simulink model "LQI_MIMO_2017a"  (R2017a)
settings: Solver=VariableStepAuto  StartTime=0.0  StopTime=4  RelTol=1e-3
values from neighbouring files (symbols this model uses):
  Klqi = lqi(sis,Q,R)    [ControladorMotor.m]    (also in ventilador.m = [Klqi Klqi(end)])
  Ts = 0.01    [ventilador.m]
undefined symbols (not defined in the file or in its folder): A, B, C
settings Model: Creator=jacqu  LastModifiedBy=Gaby
settings SFSimCC: SimUseLocalCustomCode=on
settings RTWCC: RTWUseLocalCustomCode=on

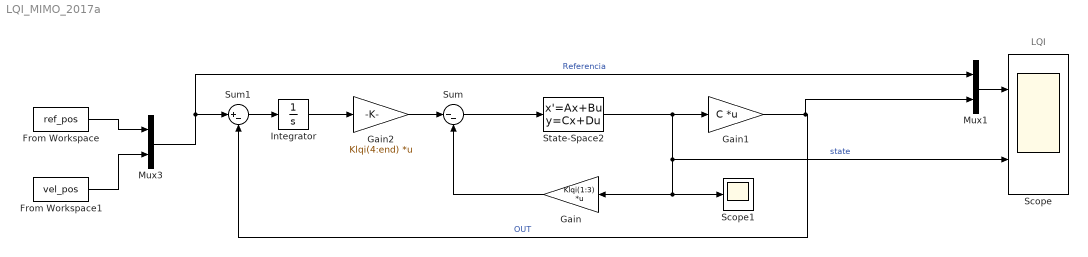
== system LQI_MIMO_2017a ==
  note: LQI
  From Workspace : FromWorkspace  VariableName=ref_pos  SampleTime=Ts
  From Workspace1 : FromWorkspace  VariableName=vel_pos  SampleTime=Ts
  Gain : Gain  Gain=Klqi(1:3)  Multiplication=Matrix(K*u) (u vector)
  Gain1 : Gain  Gain=C  Multiplication=Matrix(K*u) (u vector)
  Gain2 : Gain  Gain=Klqi(4:end)  Multiplication=Matrix(K*u) (u vector)
  Integrator : Integrator
  Mux1 : Mux  Inputs=2
  Mux3 : Mux  Inputs=2
  Scope : Scope  NumInputPorts=2
  Scope1 : Scope
  State-Space2 : StateSpace  A=A  B=B  C=eye(3)  D=zeros(3,1)  X0=0
  Sum : Sum  Inputs=|--
  Sum1 : Sum  Inputs=|+-
  wires:
  Mux3/1 -> Mux1/1, Sum1/1  "Referencia"
  Gain/1 -> Sum/2
  Gain1/1 -> Mux1/2, Sum1/2  "OUT"
  Sum/1 -> State-Space2/1
  Sum1/1 -> Integrator/1
  Integrator/1 -> Gain2/1
  Gain2/1 -> Sum/1
  State-Space2/1 -> Scope/2, Gain/1, Scope1/1, Gain1/1  "state"
  Mux1/1 -> Scope/1
  From Workspace/1 -> Mux3/1
  From Workspace1/1 -> Mux3/2
